simulink model "lab12questao3"  (Simulink 6.6)
settings: Solver=ode45  StartTime=0.0  StopTime=100.0  RelTol=1e-3
InitFcn:
  | K = 11700;
  | 
  | N = [1 1];
  | D = conv(conv([1 -1], [1 -1]), conv([1 20] ,[1 20]));
settings Model: Creator=Adriano  LastModifiedBy=Adriano

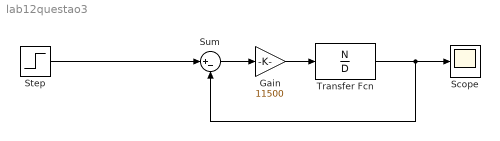
== system lab12questao3 ==
  Gain : Gain  Gain=11500
  Scope : Scope
  Step : Step  Time=0  SampleTime=0
  Sum : Sum  Inputs=|+-
  Transfer Fcn : TransferFcn  Numerator=N  Denominator=D
  wires:
  Step/1 -> Sum/1
  Sum/1 -> Gain/1
  Gain/1 -> Transfer Fcn/1
  Transfer Fcn/1 -> Sum/2, Scope/1
